simulink model "MicrogridControl"  (R2025b)
settings: Solver=VariableStepAuto  StartTime=0.0  StopTime=8  FixedStep=Ts  RelTol=1e-3
PreLoadFcn:
  | NormalOperation;
  | MicrogridControlParam;
undefined symbols (not defined in the file): base, bessModeInitial, bessSystem, bessVoltage, breakerStatus, DiscIntNeverNeededParam, ee_sli_rtmsupport, event, gcbh, generator, gflInverter, gfmInverter, Inertia, lineInductance, lineResistance, machine, plannedIsland, pmsm, powerLimit, powerQuality, PV, PVInverter, ref, resync, solar, solarInsolationChange, systemFrequency, Ts, windController, windSystem, windTurbine
libraries: nesl_utility x234, ee_lib x174, fl_lib x143, eeGeneralControl x137, simulink x78, eeTransforms x47, slpidlib x23, nesl_utility_internal x12, eePwmGenerator x9, eeSinusoidalMeasurementV2 x9, custom_lib x7, batteryecm_lib x6
(part 7 of 25)

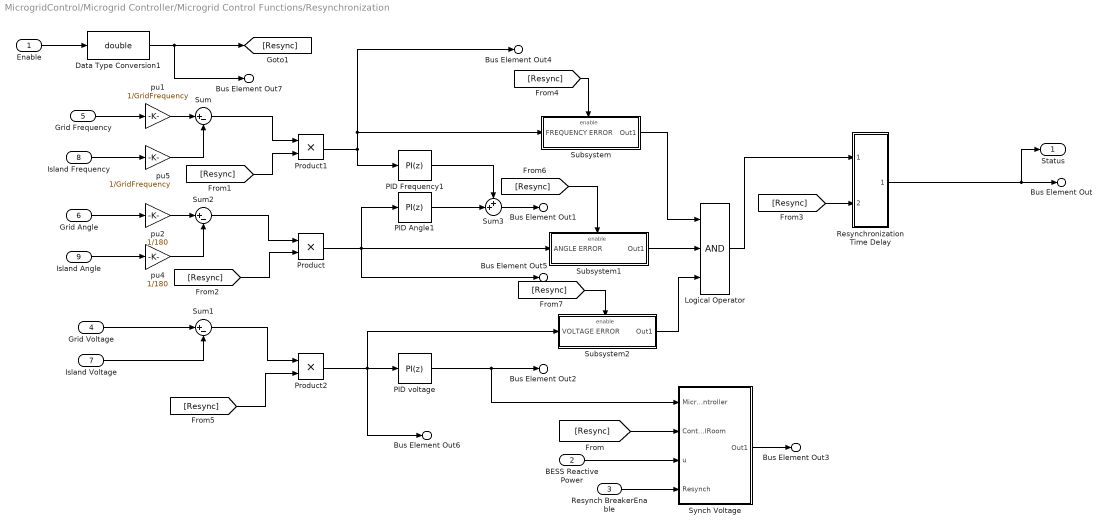
== system MicrogridControl/Microgrid Controller/Microgrid Control Functions/Resynchronization ==
  Enable : Inport
  BESS Reactive Power : Inport  Port=2
  Resynch BreakerEnable : Inport  Port=3
  Grid Voltage : Inport  Port=4
  Grid Frequency : Inport  Port=5
  Grid Angle : Inport  Port=6
  Island Voltage : Inport  Port=7
  Island Frequency : Inport  Port=8
  Island Angle : Inport  Port=9
  Data Type Conversion1 : DataTypeConversion  OutDataTypeStr=double  SaturateOnIntegerOverflow=off  RndMeth=Floor
  Logical Operator : Logic  Inputs=3  AllPortsSameDT=off  OutDataTypeStr=boolean
  PID Angle1 : slpidlib/PID Controller  Controller=PI  Form=Parallel  TimeDomain=Discrete-time  UseExternalTs=off  SampleTime=Ts  IntegratorMethod=Forward Euler  FilterMethod=Forward Euler  ControllerParametersSource=internal  P=KpAngResynch  I=KiAngResynch  UseKiTs=off  D=0  UseExternalDerivativeSource=off  N=100  UseFilter=on  TunerSelectOption=Frequency Response Based  InitialConditionSource=internal  InitialConditionForIntegrator=0  InitialConditionForFilter=0  DifferentiatorICPrevScaledInput=0  ExternalReset=none  TrackingMode=off  Kt=1  LimitOutput=off  SatLimitsSource=internal  UpperSaturationLimit=0.5  LowerSaturationLimit=-0.5  LinearizeAsGain=on  AntiWindupMode=clamping  Kb=1  LimitIntegrator=off  UpperIntegratorSaturationLimit=inf  LowerIntegratorSaturationLimit=-inf  POutMin=[]  POutMax=[]  IOutMin=[]  IOutMax=[]  DOutMin=[]  DOutMax=[]  NOutMin=[]  NOutMax=[]  SumOutMin=[]  SumOutMax=[]  SaturationOutMin=[]  SaturationOutMax=[]  PParamMin=[]  PParamMax=[]  IParamMin=[]  IParamMax=[]  DParamMin=[]  DParamMax=[]  NParamMin=[]  NParamMax=[]  KbParamMin=[]  KbParamMax=[]  KtParamMin=[]  KtParamMax=[]  KbOutMin=[]  KbOutMax=[]  KtOutMin=[]  KtOutMax=[]  IntegratorOutMin=[]  IntegratorOutMax=[]  FilterOutMin=[]  FilterOutMax=[]  SumI1OutMin=[]  SumI1OutMax=[]  SumI2OutMin=[]  SumI2OutMax=[]  SumI3OutMin=[]  SumI3OutMax=[]  SumI4OutMin=[]  SumI4OutMax=[]  SumDOutMin=[]  SumDOutMax=[]  DifferentiatorOutMin=[]  DifferentiatorOutMax=[]  FilterDiffOutCoefMin=[]  FilterDiffOutCoefMax=[]  ReciprocalOutMin=[]  ReciprocalOutMax=[]  SumDenOutMin=[]  SumDenOutMax=[]  SumNumOutMin=[]  SumNumOutMax=[]  DivideOutMin=[]  DivideOutMax=[]  UdiffTsProdOutMin=[]  UdiffTsProdOutMax=[]  NTsProdOutMin=[]  NTsProdOutMax=[]  UintegralTsProdOutMin=[]  UintegralTsProdOutMax=[]  UngainTsProdOutMin=[]  UngainTsProdOutMax=[]  ClampingZeroOutDataTypeStr=Inherit: Inherit via back propagation  ClampingZeroOutMin=[]  ClampingZeroOutMax=[]  FilterDenConstantOutDataTypeStr=Inherit: Inherit via back propagation  FilterDenConstantOutMin=[]  FilterDenConstantOutMax=[]  PCopyOutDataTypeStr=Inherit: Inherit via back propagation  PCopyOutMin=[]  PCopyOutMax=[]  NCopyOutDataTypeStr=Inherit: Inherit via back propagation  NCopyOutMin=[]  NCopyOutMax=[]  IntegratorContinuousStateAttributes=''  IntegratorStateMustResolveToSignalObject=off  IntegratorRTWStateStorageClass=Auto  FilterContinuousStateAttributes=''  FilterStateMustResolveToSignalObject=off  FilterRTWStateStorageClass=Auto  ParallelPVariant=InternalParameters  IdealPVariant=Disabled  IVariant=InternalParameters  DVariant=Disabled  IntegratorVariant=Discrete  SatVariant=Disabled  AWVariant=Passthrough  PCopyVariant=Disabled  TRVariant=Disabled  FdbkBlocksVariant=Forward  IdealPFdbkVariant=Disabled  SatFdbkVariant=Disabled  DerivativeFilterVariant=Disabled  NVariant=Disabled  NCopyVariant=Disabled_SignalSpec  FilterICVariant=Disabled  IntegratorICVariant=InternalICs  ExternalResetVariant=Disabled  TRSumVariant=Passthrough  SumFdbkVariant=Disabled  SumVariant=Sum_PI  TsampFilterVariant=InternalTs  TsampNgainVariant=Passthrough  TsampIntegralVariant=Disabled_SignalSpec  ExternalSaturationOutDataTypeStr=Inherit: Same as second input  DerivativeSourceVariant=Disabled  PreIntVariant=InternalPreInt
  PID Frequency1 : slpidlib/PID Controller  Controller=PI  Form=Parallel  TimeDomain=Discrete-time  UseExternalTs=off  SampleTime=Ts  IntegratorMethod=Forward Euler  FilterMethod=Forward Euler  ControllerParametersSource=internal  P=KpFreResynch  I=KiFreResynch  UseKiTs=off  D=0  UseExternalDerivativeSource=off  N=100  UseFilter=on  TunerSelectOption=Frequency Response Based  InitialConditionSource=internal  InitialConditionForIntegrator=0  InitialConditionForFilter=0  DifferentiatorICPrevScaledInput=0  ExternalReset=none  TrackingMode=off  Kt=1  LimitOutput=off  SatLimitsSource=internal  UpperSaturationLimit=0.05  LowerSaturationLimit=-0.05  LinearizeAsGain=on  AntiWindupMode=clamping  Kb=1  LimitIntegrator=off  UpperIntegratorSaturationLimit=inf  LowerIntegratorSaturationLimit=-inf  POutMin=[]  POutMax=[]  IOutMin=[]  IOutMax=[]  DOutMin=[]  DOutMax=[]  NOutMin=[]  NOutMax=[]  SumOutMin=[]  SumOutMax=[]  SaturationOutMin=[]  SaturationOutMax=[]  PParamMin=[]  PParamMax=[]  IParamMin=[]  IParamMax=[]  DParamMin=[]  DParamMax=[]  NParamMin=[]  NParamMax=[]  KbParamMin=[]  KbParamMax=[]  KtParamMin=[]  KtParamMax=[]  KbOutMin=[]  KbOutMax=[]  KtOutMin=[]  KtOutMax=[]  IntegratorOutMin=[]  IntegratorOutMax=[]  FilterOutMin=[]  FilterOutMax=[]  SumI1OutMin=[]  SumI1OutMax=[]  SumI2OutMin=[]  SumI2OutMax=[]  SumI3OutMin=[]  SumI3OutMax=[]  SumI4OutMin=[]  SumI4OutMax=[]  SumDOutMin=[]  SumDOutMax=[]  DifferentiatorOutMin=[]  DifferentiatorOutMax=[]  FilterDiffOutCoefMin=[]  FilterDiffOutCoefMax=[]  ReciprocalOutMin=[]  ReciprocalOutMax=[]  SumDenOutMin=[]  SumDenOutMax=[]  SumNumOutMin=[]  SumNumOutMax=[]  DivideOutMin=[]  DivideOutMax=[]  UdiffTsProdOutMin=[]  UdiffTsProdOutMax=[]  NTsProdOutMin=[]  NTsProdOutMax=[]  UintegralTsProdOutMin=[]  UintegralTsProdOutMax=[]  UngainTsProdOutMin=[]  UngainTsProdOutMax=[]  ClampingZeroOutDataTypeStr=Inherit: Inherit via back propagation  ClampingZeroOutMin=[]  ClampingZeroOutMax=[]  FilterDenConstantOutDataTypeStr=Inherit: Inherit via back propagation  FilterDenConstantOutMin=[]  FilterDenConstantOutMax=[]  PCopyOutDataTypeStr=Inherit: Inherit via back propagation  PCopyOutMin=[]  PCopyOutMax=[]  NCopyOutDataTypeStr=Inherit: Inherit via back propagation  NCopyOutMin=[]  NCopyOutMax=[]  IntegratorContinuousStateAttributes=''  IntegratorStateMustResolveToSignalObject=off  IntegratorRTWStateStorageClass=Auto  FilterContinuousStateAttributes=''  FilterStateMustResolveToSignalObject=off  FilterRTWStateStorageClass=Auto  ParallelPVariant=InternalParameters  IdealPVariant=Disabled  IVariant=InternalParameters  DVariant=Disabled  IntegratorVariant=Discrete  SatVariant=Disabled  AWVariant=Passthrough  PCopyVariant=Disabled  TRVariant=Disabled  FdbkBlocksVariant=Forward  IdealPFdbkVariant=Disabled  SatFdbkVariant=Disabled  DerivativeFilterVariant=Disabled  NVariant=Disabled  NCopyVariant=Disabled_SignalSpec  FilterICVariant=Disabled  IntegratorICVariant=InternalICs  ExternalResetVariant=Disabled  TRSumVariant=Passthrough  SumFdbkVariant=Disabled  SumVariant=Sum_PI  TsampFilterVariant=InternalTs  TsampNgainVariant=Passthrough  TsampIntegralVariant=Disabled_SignalSpec  ExternalSaturationOutDataTypeStr=Inherit: Same as second input  DerivativeSourceVariant=Disabled  PreIntVariant=InternalPreInt
  PID voltage : slpidlib/PID Controller  Controller=PI  Form=Parallel  TimeDomain=Discrete-time  UseExternalTs=off  SampleTime=Ts  IntegratorMethod=Forward Euler  FilterMethod=Forward Euler  ControllerParametersSource=internal  P=KpVolResynch  I=KiVolResynch  UseKiTs=off  D=0  UseExternalDerivativeSource=off  N=100  UseFilter=on  TunerSelectOption=Frequency Response Based  InitialConditionSource=internal  InitialConditionForIntegrator=1  InitialConditionForFilter=0  DifferentiatorICPrevScaledInput=0  ExternalReset=none  TrackingMode=off  Kt=1  LimitOutput=off  SatLimitsSource=internal  UpperSaturationLimit=1.5  LowerSaturationLimit=-0.05  LinearizeAsGain=on  AntiWindupMode=clamping  Kb=1  LimitIntegrator=off  UpperIntegratorSaturationLimit=inf  LowerIntegratorSaturationLimit=-inf  POutMin=[]  POutMax=[]  IOutMin=[]  IOutMax=[]  DOutMin=[]  DOutMax=[]  NOutMin=[]  NOutMax=[]  SumOutMin=[]  SumOutMax=[]  SaturationOutMin=[]  SaturationOutMax=[]  PParamMin=[]  PParamMax=[]  IParamMin=[]  IParamMax=[]  DParamMin=[]  DParamMax=[]  NParamMin=[]  NParamMax=[]  KbParamMin=[]  KbParamMax=[]  KtParamMin=[]  KtParamMax=[]  KbOutMin=[]  KbOutMax=[]  KtOutMin=[]  KtOutMax=[]  IntegratorOutMin=[]  IntegratorOutMax=[]  FilterOutMin=[]  FilterOutMax=[]  SumI1OutMin=[]  SumI1OutMax=[]  SumI2OutMin=[]  SumI2OutMax=[]  SumI3OutMin=[]  SumI3OutMax=[]  SumI4OutMin=[]  SumI4OutMax=[]  SumDOutMin=[]  SumDOutMax=[]  DifferentiatorOutMin=[]  DifferentiatorOutMax=[]  FilterDiffOutCoefMin=[]  FilterDiffOutCoefMax=[]  ReciprocalOutMin=[]  ReciprocalOutMax=[]  SumDenOutMin=[]  SumDenOutMax=[]  SumNumOutMin=[]  SumNumOutMax=[]  DivideOutMin=[]  DivideOutMax=[]  UdiffTsProdOutMin=[]  UdiffTsProdOutMax=[]  NTsProdOutMin=[]  NTsProdOutMax=[]  UintegralTsProdOutMin=[]  UintegralTsProdOutMax=[]  UngainTsProdOutMin=[]  UngainTsProdOutMax=[]  ClampingZeroOutDataTypeStr=Inherit: Inherit via back propagation  ClampingZeroOutMin=[]  ClampingZeroOutMax=[]  FilterDenConstantOutDataTypeStr=Inherit: Inherit via back propagation  FilterDenConstantOutMin=[]  FilterDenConstantOutMax=[]  PCopyOutDataTypeStr=Inherit: Inherit via back propagation  PCopyOutMin=[]  PCopyOutMax=[]  NCopyOutDataTypeStr=Inherit: Inherit via back propagation  NCopyOutMin=[]  NCopyOutMax=[]  IntegratorContinuousStateAttributes=''  IntegratorStateMustResolveToSignalObject=off  IntegratorRTWStateStorageClass=Auto  FilterContinuousStateAttributes=''  FilterStateMustResolveToSignalObject=off  FilterRTWStateStorageClass=Auto  ParallelPVariant=InternalParameters  IdealPVariant=Disabled  IVariant=InternalParameters  DVariant=Disabled  IntegratorVariant=Discrete  SatVariant=Disabled  AWVariant=Passthrough  PCopyVariant=Disabled  TRVariant=Disabled  FdbkBlocksVariant=Forward  IdealPFdbkVariant=Disabled  SatFdbkVariant=Disabled  DerivativeFilterVariant=Disabled  NVariant=Disabled  NCopyVariant=Disabled_SignalSpec  FilterICVariant=Disabled  IntegratorICVariant=InternalICs  ExternalResetVariant=Disabled  TRSumVariant=Passthrough  SumFdbkVariant=Disabled  SumVariant=Sum_PI  TsampFilterVariant=InternalTs  TsampNgainVariant=Passthrough  TsampIntegralVariant=Disabled_SignalSpec  ExternalSaturationOutDataTypeStr=Inherit: Same as second input  DerivativeSourceVariant=Disabled  PreIntVariant=InternalPreInt
  Product : Product
  Product1 : Product
  Product2 : Product
  Resynchronization Time Delay : Subsystem
  Subsystem : Subsystem
  Subsystem1 : Subsystem
  Subsystem2 : Subsystem
  Sum : Sum  Inputs=|+-
  Sum1 : Sum  Inputs=|+-
  Sum2 : Sum  Inputs=|+-
  Sum3 : Sum  Inputs=++|
  Synch Voltage : Subsystem
  pu1 : Gain  Gain=1/GridFrequency
  pu2 : Gain  Gain=1/180
  pu4 : Gain  Gain=1/180
  pu5 : Gain  Gain=1/GridFrequency
  Status : Outport
  Bus Element Out : Outport  Port=2  PortName=Resync  Element=status
  Bus Element Out1 : Outport  Port=2  PortName=Resync  Element=synchFrequency
  Bus Element Out2 : Outport  Port=2  PortName=Resync  Element=synchVoltage
  Bus Element Out3 : Outport  Port=2  PortName=Resync  Element=synchVoltagedpr
  Bus Element Out4 : Outport  Port=2  PortName=Resync  Element=frequencyerror
  Bus Element Out5 : Outport  Port=2  PortName=Resync  Element=phasError
  Bus Element Out6 : Outport  Port=2  PortName=Resync  Element=voltageMagError
  Bus Element Out7 : Outport  Port=2  PortName=Resync  Element=enableCommand
  wires:
  PID Frequency1/1 -> Sum3/1
  pu1/1 -> Sum/1
  Resynch BreakerEnable/1 -> Synch Voltage/4(Resynch)
  Island Voltage/1 -> Sum1/2
  Product1/1 -> Bus Element Out4/1, Subsystem/1(FREQUENCY ERROR), PID Frequency1/1
  Sum2/1 -> Product/1
  pu4/1 -> Sum2/2
  BESS Reactive Power/1 -> Synch Voltage/3(u)
  PID Angle1/1 -> Sum3/2
  Island Frequency/1 -> pu5/1
  pu2/1 -> Sum2/1
  Data Type Conversion1/1 -> Bus Element Out7/1, [Resync]
  Product2/1 -> PID voltage/1, Bus Element Out6/1, Subsystem2/1(VOLTAGE ERROR)
  Grid Voltage/1 -> Sum1/1
  Island Angle/1 -> pu4/1
  [Resync] -> Product1/2
  Grid Angle/1 -> pu2/1
  Grid Frequency/1 -> pu1/1
  Product/1 -> Bus Element Out5/1, Subsystem1/1(ANGLE ERROR), PID Angle1/1
  Subsystem/1(Out1) -> Logical Operator/1
  Resynchronization Time Delay/1(MGController) -> Bus Element Out/1, Status/1
  pu5/1 -> Sum/2
  [Resync] -> Product2/2
  [Resync] -> Resynchronization Time Delay/2(In2)
  Logical Operator/1 -> Resynchronization Time Delay/1(In1)
  [Resync] -> Synch Voltage/2(ControlRoom)
  Subsystem2/1(Out1) -> Logical Operator/3
  Subsystem1/1(Out1) -> Logical Operator/2
  [Resync] -> Subsystem2/Enable
  Synch Voltage/1(Out1) -> Bus Element Out3/1
  Sum1/1 -> Product2/1
  Enable/1 -> Data Type Conversion1/1
  Sum3/1 -> Bus Element Out1/1
  Sum/1 -> Product1/1
  PID voltage/1 -> Bus Element Out2/1, Synch Voltage/1(MicrogridController)
  [Resync] -> Subsystem/Enable
  [Resync] -> Product/2
  [Resync] -> Subsystem1/Enable

== system MicrogridControl/Microgrid Controller/Microgrid Supervisory Control/Transition and Dispatch Control/On.Black_Start ==
  blackStartComplete : Inport
  blackStartEnable : Inport  Port=2
  " Demux " : Demux  Outputs=1
  " SFunction " : S-Function  Tag=Stateflow S-Function 8  FunctionName=sf_sfun  PortCounts=[2 3]  SFunctionDeploymentMode=off  EnableBusSupport=off
  " Terminator " : Terminator
  blackStartStatus : Outport
  blackStart : Outport  Port=2
  wires:
  blackStartComplete/1 -> " SFunction "/1
  blackStartEnable/1 -> " SFunction "/2
  " SFunction "/2 -> blackStartStatus/1  "blackStartStatus"
  " SFunction "/3 -> blackStart/1  "blackStart"
  " Demux "/1 -> " Terminator "/1
  " SFunction "/1 -> " Demux "/1

== system MicrogridControl/Microgrid Controller/Microgrid Supervisory Control/Transition and Dispatch Control/On.Planned_Islanding ==
  PlannedIslanding : Inport
  " Demux " : Demux  Outputs=1
  " SFunction " : S-Function  Tag=Stateflow S-Function 18  FunctionName=sf_sfun  PortCounts=[1 6]  SFunctionDeploymentMode=off  EnableBusSupport=off
  " Terminator " : Terminator
  PCC : Outport
  plannedIslanding : Outport  Port=2
  plannedIslandingStatus : Outport  Port=3
  mode : Outport  Port=4
  motorBreaker : Outport  Port=5
  wires:
  PlannedIslanding/1 -> " SFunction "/1
  " SFunction "/2 -> PCC/1  "PCC"
  " SFunction "/3 -> plannedIslanding/1  "plannedIslanding"
  " SFunction "/4 -> plannedIslandingStatus/1  "plannedIslandingStatus"
  " SFunction "/5 -> mode/1  "mode"
  " SFunction "/6 -> motorBreaker/1  "motorBreaker"
  " Demux "/1 -> " Terminator "/1
  " SFunction "/1 -> " Demux "/1

== system MicrogridControl/Microgrid Controller/Microgrid Supervisory Control/Transition and Dispatch Control/On.Resynchronization ==
  Resync : Inport
  " Demux " : Demux  Outputs=1
  " SFunction " : S-Function  Tag=Stateflow S-Function 19  FunctionName=sf_sfun  PortCounts=[1 5]  SFunctionDeploymentMode=off  EnableBusSupport=off
  " Terminator " : Terminator
  PCC : Outport
  resync : Outport  Port=2
  resyncStatus : Outport  Port=3
  mode : Outport  Port=4
  wires:
  Resync/1 -> " SFunction "/1
  " SFunction "/2 -> PCC/1  "PCC"
  " SFunction "/3 -> resync/1  "resync"
  " SFunction "/4 -> resyncStatus/1  "resyncStatus"
  " SFunction "/5 -> mode/1  "mode"
  " Demux "/1 -> " Terminator "/1
  " SFunction "/1 -> " Demux "/1

== system MicrogridControl/Microgrid Controller/Microgrid Supervisory Control/Transition and Dispatch Control/On.Steady_State_Grid_Connected ==
  " Demux " : Demux  Outputs=1
  " Ground " : Ground
  " SFunction " : S-Function  Tag=Stateflow S-Function 20  FunctionName=sf_sfun  PortCounts=[1 3]  SFunctionDeploymentMode=off  EnableBusSupport=off
  " Terminator " : Terminator
  emergencyDispatch : Outport
  mode : Outport  Port=2
  wires:
  " SFunction "/2 -> emergencyDispatch/1  "emergencyDispatch"
  " SFunction "/3 -> mode/1  "mode"
  " Ground "/1 -> " SFunction "/1
  " Demux "/1 -> " Terminator "/1
  " SFunction "/1 -> " Demux "/1

== system MicrogridControl/Microgrid Controller/Microgrid Supervisory Control/Transition and Dispatch Control/On.Steady_State_Islanded ==
  plannedIslandingDispatch : Inport
  " Demux " : Demux  Outputs=1
  " SFunction " : S-Function  Tag=Stateflow S-Function 21  FunctionName=sf_sfun  PortCounts=[1 3]  SFunctionDeploymentMode=off  EnableBusSupport=off
  " Terminator " : Terminator
  emergencyDispatch : Outport
  motorBreaker : Outport  Port=2
  wires:
  plannedIslandingDispatch/1 -> " SFunction "/1
  " SFunction "/2 -> emergencyDispatch/1  "emergencyDispatch"
  " SFunction "/3 -> motorBreaker/1  "motorBreaker"
  " Demux "/1 -> " Terminator "/1
  " SFunction "/1 -> " Demux "/1

== system MicrogridControl/Microgrid Controller/Microgrid Supervisory Control/Transition and Dispatch Control/On.Unplanned_Islanding ==
  " Demux " : Demux  Outputs=1
  " Ground " : Ground
  " SFunction " : S-Function  Tag=Stateflow S-Function 22  FunctionName=sf_sfun  PortCounts=[1 3]  SFunctionDeploymentMode=off  EnableBusSupport=off
  " Terminator " : Terminator
  PCC : Outport
  emergencyDispatch : Outport  Port=2
  wires:
  " SFunction "/2 -> PCC/1  "PCC"
  " SFunction "/3 -> emergencyDispatch/1  "emergencyDispatch"
  " Ground "/1 -> " SFunction "/1
  " Demux "/1 -> " Terminator "/1
  " SFunction "/1 -> " Demux "/1

== system MicrogridControl/Microgrid Controller/Reference Generation/Active and Reactive Powers ==
  Planned Islanding : Inport
  Planned Islanding PRef : Inport  Port=2
  Planned Islanding QRef : Inport  Port=3
  Control Room PRef : Inport  Port=4
  Control Room QRef : Inport  Port=5
  Saturation : Saturate  UpperLimit=1  LowerLimit=-1
  Saturation1 : Saturate  UpperLimit=1  LowerLimit=-1
  Sum : Sum  Inputs=|++
  Sum1 : Sum  Inputs=|++
  Switch : Switch  Criteria=u2 > Threshold  Threshold=0.5  SaturateOnIntegerOverflow=off  InputSameDT=off
  Switch1 : Switch  Criteria=u2 > Threshold  Threshold=0.5  SaturateOnIntegerOverflow=off  InputSameDT=off
  PRef : Outport
  QRef : Outport  Port=2
  wires:
  Saturation1/1 -> QRef/1
  Saturation/1 -> PRef/1
  Switch/1 -> Saturation/1  "Pref"
  Sum/1 -> Switch/1
  Switch1/1 -> Saturation1/1  "Qref"
  Sum1/1 -> Switch1/1
  Control Room PRef/1 -> Switch/3, Sum/2
  Control Room QRef/1 -> Sum1/2, Switch1/3
  Planned Islanding/1 -> Switch1/2, Switch/2
  Planned Islanding PRef/1 -> Sum/1
  Planned Islanding QRef/1 -> Sum1/1

== system MicrogridControl/Microgrid Controller/Reference Generation/Frequency ==
  Reference Island Frequency : Inport
  Resynch Command : Inport  Port=2
  Power command : Inport  Port=3
  Resych Frequency : Inport  Port=4
  Black Start : Inport  Port=5
  Black Start Frequency : Inport  Port=6
  Constant1 : Constant  Value=1%frequencyPLL
  Scope : Scope  NumInputPorts=2
      settings: ActiveDisplayYMinimum=-1  ActiveDisplayYMaximum=1  DataLoggingVariableName=ScopeData2
  Scope1 : Scope  NumInputPorts=3
      settings: ActiveDisplayYMinimum=-1  ActiveDisplayYMaximum=1  DataLoggingVariableName=ScopeData3
  Sum : Sum  Inputs=|++
  Switch : Switch  Criteria=u2 > Threshold  Threshold=0.5  SaturateOnIntegerOverflow=off  InputSameDT=off
  Switch1 : Switch  Criteria=u2 > Threshold  Threshold=0.5  SaturateOnIntegerOverflow=off  InputSameDT=off
  Switch2 : Switch  Criteria=u2 > Threshold  Threshold=0.5  SaturateOnIntegerOverflow=off  InputSameDT=off
  FRef : Outport
  wires:
  Switch2/1 -> Switch1/3
  Resych Frequency/1 -> Sum/1
  Black Start Frequency/1 -> Scope1/3, Switch1/1
  Black Start/1 -> Scope1/1, Switch1/2
  Power command/1 -> Switch2/2
  Reference Island Frequency/1 -> Sum/2, Switch/3
  Sum/1 -> Scope/2, Switch/1
  Constant1/1 -> Switch2/1
  Switch/1 -> Switch2/3
  Resynch Command/1 -> Scope/1, Switch/2
  Switch1/1 -> FRef/1, Scope1/2

== system MicrogridControl/Microgrid Controller/Reference Generation/Voltage ==
  Reference Island Voltage : Inport
  Resynch Voltage : Inport  Port=2
  Resynch Command : Inport  Port=3
  Blackstart Command : Inport  Port=4
  Black Start voltage : Inport  Port=5
  Scope : Scope  NumInputPorts=2
      settings: ActiveDisplayYMinimum=-1  ActiveDisplayYMaximum=1
  Scope1 : Scope  NumInputPorts=2
      settings: ActiveDisplayYMinimum=-1  ActiveDisplayYMaximum=1
  Switch1 : Switch  Criteria=u2 > Threshold  Threshold=0.5  SaturateOnIntegerOverflow=off  InputSameDT=off
  Switch2 : Switch  Criteria=u2 > Threshold  Threshold=0.5  SaturateOnIntegerOverflow=off  InputSameDT=off
  VRef : Outport
  wires:
  Switch2/1 -> Scope1/2, VRef/1
  Switch1/1 -> Switch2/3
  Reference Island Voltage/1 -> Scope/1, Switch1/3
  Blackstart Command/1 -> Scope1/1, Switch2/2
  Black Start voltage/1 -> Switch2/1
  Resynch Voltage/1 -> Switch1/1
  Resynch Command/1 -> Scope/2, Switch1/2

== system MicrogridControl/Microgrid Controller/Subsystem1/PLL ==
  abc : Inport
  Frequency Measurement : Subsystem
  Gain : Gain  Gain=1/sqrt(2)
  "Sinusoidal Measurement (PLL, Three-Phase)" : eeSinusoidalMeasurement/Sinusoidal Measurement (PLL, Three-Phase)  Kp_LF=40  Ki_LF=1000  F0=50  Theta0=0  Ts=-1
  Subsystem : Subsystem
  fre : Outport
  angle : Outport  Port=2
  mag : Outport  Port=3
  wires:
  abc/1 -> Frequency Measurement/1(Vabc), "Sinusoidal Measurement (PLL, Three-Phase)"/1
  "Sinusoidal Measurement (PLL, Three-Phase)"/3 -> Gain/1
  "Sinusoidal Measurement (PLL, Three-Phase)"/2 -> Subsystem/1(In)
  Subsystem/1(Out) -> angle/1
  Gain/1 -> mag/1
  Frequency Measurement/1(freq) -> fre/1

== system MicrogridControl/Microgrid Controller/Subsystem1/PLL start at 0.2 s ==
  PCC measurement : Inport
  Constant : Constant  Value=0
  Step : Step  Time=0.2  SampleTime=Ts
  Switch : Switch  Criteria=u2 > Threshold  Threshold=0.5  SaturateOnIntegerOverflow=off  InputSameDT=off
  Out1 : Outport
  wires:
  PCC measurement/1 -> Switch/1
  Switch/1 -> Out1/1
  Constant/1 -> Switch/3
  Step/1 -> Switch/2

== system MicrogridControl/Microgrid Controller/Subsystem1/PLL starts at 0.2 s ==
  PCC measurement : Inport
  Constant1 : Constant  Value=0
  Step : Step  Time=0.2  SampleTime=Ts
  Switch : Switch  Criteria=u2 > Threshold  Threshold=0.5  SaturateOnIntegerOverflow=off  InputSameDT=off
  abc : Outport
  wires:
  PCC measurement/1 -> Switch/1
  Constant1/1 -> Switch/3
  Switch/1 -> abc/1
  Step/1 -> Switch/2

== system MicrogridControl/Microgrid Controller/Subsystem1/PLL1 ==
  abc : Inport
  Frequency Measurement : Subsystem
  Gain : Gain  Gain=1/sqrt(2)
  "Sinusoidal Measurement (PLL, Three-Phase)" : eeSinusoidalMeasurement/Sinusoidal Measurement (PLL, Three-Phase)  Kp_LF=40  Ki_LF=1000  F0=50  Theta0=0  Ts=-1
  Subsystem : Subsystem
  fre : Outport
  angle : Outport  Port=2
  mag : Outport  Port=3
  wires:
  abc/1 -> Frequency Measurement/1(Vabc), "Sinusoidal Measurement (PLL, Three-Phase)"/1
  "Sinusoidal Measurement (PLL, Three-Phase)"/3 -> Gain/1
  "Sinusoidal Measurement (PLL, Three-Phase)"/2 -> Subsystem/1(In)
  Subsystem/1(Out) -> angle/1
  Gain/1 -> mag/1
  Frequency Measurement/1(freq) -> fre/1

== system MicrogridControl/Motor Load/Motor Loads/Subsystem ==
  Gain : Gain  Commented=on  Gain=60/(2*pi)
  Ideal Rotational Motion Sensor : fl_lib/Mechanical/Mechanical Sensors/Ideal Rotational Motion Sensor  Commented=on  reference=foundation.enum.MeasurementReference.difference  acceleration_port=false  velocity_port=true  position_port=false  wrap_angle=false  offset=0 rad
      settings: InternalSimscapePortConfiguration="{\"Bottom\":[],\"Left\":[{\"id\":\"R\",\"label\":\"R\",\"type\":\"foundation.mechanical.rotational.rotational\"}],\"Right\":[{\"id\":\"C\",\"label\":\"C\",\"type\":\"foundation.mechanical.rotational.rotational\"},{\"id\":\"W\",\"label\":\"W\",\"type\":\"output\"}],\"Top\":[]}"
  Ideal Torque Source : fl_lib/Mechanical/Mechanical Sources/Ideal Torque Source
  Mechanical Rotational Reference : fl_lib/Mechanical/Rotational Elements/Mechanical Rotational Reference
  PS Constant : fl_lib/Physical Signals/Sources/PS Constant  Commented=on  constant=300000
  PS Step : fl_lib/Physical Signals/Sources/PS Step  step_time=0.1 s  initial_value=0  final_value=-9000
  PS-Simulink Converter : nesl_utility/PS-Simulink Converter  Commented=on  PhysicalDomain=network_engine_domain  SubClassName=ps_output  LeftPortType=input  RightPortType=output  PseudoPeriodic=off  Frequencies=[]  VectorFormat=inherit  Unit=inherit  AffineConversion=off
  Rotational Friction : fl_lib/Mechanical/Rotational Elements/Rotational Friction  brkwy_trq=25 N*m  brkwy_vel=0.1 rad/s  Col_trq=20 N*m  visc_coef=0.001 N*m*s/rad  w_specify=on  w_priority=None  w=0 rad/s  w_nominal_specify=off  w_nominal_value=1  w_nominal_unit=rad/s  t_specify=on  t_priority=None  t=0 N*m  t_nominal_specify=off  t_nominal_value=1  t_nominal_unit=N*m
  Scope : Scope  Commented=on
      settings: ActiveDisplayYMinimum=566.67789  ActiveDisplayYMaximum=1937.03579
  Step : Step  Commented=on  Time=0.05  After=300000  SampleTime=0
  Conn1 : PMIOPort  Side=Left
  Conn2 : PMIOPort  Port=2  Side=Left
  wires:
  Gain/1 -> Scope/1
  PS-Simulink Converter/1 -> Gain/1
  connections:
  Rotational Friction/RConn1 -- Ideal Rotational Motion Sensor/RConn1 -- Conn2/RConn1 -- Mechanical Rotational Reference/LConn1 -- Ideal Torque Source/RConn2
  Rotational Friction/LConn1 -- Conn1/RConn1 -- Ideal Rotational Motion Sensor/LConn1 -- Ideal Torque Source/LConn1
  PS-Simulink Converter/LConn1 -- Ideal Rotational Motion Sensor/RConn2
  PS Step/RConn1 -- Ideal Torque Source/RConn1

== system MicrogridControl/Solar/Solar Plant Integrated/Detailed ==
  Ir : Inport
  T : Inport  Port=2
  Pref : Inport  Port=3
  Qref : Inport  Port=4
  Mode : Inport  Port=5
  L Filter2 : ee_lib/Passive/RLC Assemblies/RLC (Three-Phase)  port_option=ee.enum.threePhasePort.composite  component_structure=ee.enum.rlc.structure.SeriesRL  R=filterResistance Ohm  L=filterInductance H  C=1e-6 F  R_parasitic=0 Ohm  G_parasitic=0 1/Ohm  IL_specify=on  IL_priority=None  IL=[0, 0, 0] A  IL_nominal_specify=off  IL_nominal_value=1  IL_nominal_unit=A  VC_specify=off  VC_priority=High  VC=[0, 0, 0] V  VC_nominal_specify=off  VC_nominal_value=1  VC_nominal_unit=V
      settings: InternalSimscapePortConfiguration="{\"Bottom\":[],\"Left\":[{\"id\":\"N1\",\"label\":\"~1\",\"type\":\"foundation.electrical.three_phase\"}],\"Right\":[{\"id\":\"N2\",\"label\":\"~2\",\"type\":\"foundation.electrical.three_phase\"}],\"Top\":[]}"
  Measurements : Subsystem
  PV Plant & Controller : Subsystem
  Terminator : Terminator
  ~ : PMIOPort  Side=Right
  Out Bus Element23 : Outport  PortName=Meas  Element=activePower
  Out Bus Element1 : Outport  PortName=Meas  Element=reactivePower
  Out Bus Element2 : Outport  PortName=Meas  Element=voltage
  Out Bus Element3 : Outport  PortName=Meas  Element=current
  wires:
  Measurements/2(Q) -> Out Bus Element1/1
  Measurements/4(I) -> Out Bus Element3/1, PV Plant & Controller/5(Iabc)
  Qref/1 -> PV Plant & Controller/3(Qref)
  Ir/1 -> PV Plant & Controller/1(Insolation)
  Measurements/3(V) -> Out Bus Element2/1, PV Plant & Controller/4(Vabc)
  Measurements/1(P) -> Out Bus Element23/1
  T/1 -> Terminator/1
  Pref/1 -> PV Plant & Controller/2(Pref)
  Mode/1 -> PV Plant & Controller/6(Mode)
  connections:
  L Filter2/RConn1 -- Measurements/LConn1
  L Filter2/LConn1 -- PV Plant & Controller/RConn1
  Measurements/RConn1 -- ~/RConn1

== system MicrogridControl/Solar/Solar Plant Integrated/Simplified ==
  Ir : Inport
  T : Inport  Port=2
  Pref : Inport  Port=3
  Qref : Inport  Port=4
  Mode : Inport  Port=5
  Measurements : Subsystem
  Simulink-PS Converter{,1..4} (5 alike) : nesl_utility/Simulink-PS Converter  PhysicalDomain=network_engine_domain  SubClassName=ps_input  LeftPortType=input  RightPortType=output  PseudoPeriodic=off  Frequencies=[]  NoiseDistribution=none  NoiseParameters=[]  Unit=1  AffineConversion=off  FilteringAndDerivatives=provide  SimscapeFilterOrder=1  InputFilterTimeConstant=0.001  UdotUserProvided=0
  solar_plant : custom_lib/solar_plant  port_option=ee.enum.threePhasePort.composite  FRated=frequency Hz  VRated=Vac V  PlantRating=plantRating kW  modelling_option=ModellingOption.powerReference  Vdc=2*Vac*sqrt(2/3) V  IMaxPU=iMaxPU  efficiency=efficiency  IrRef=irradianceSTC W/m^2  T=temperatureSTC K  PVTech=PanelTechnology.polycrystallinePanel  PanelRating=panelRating W  VocRef=Voc V  IscRef=Isc A  alpha=alpha 1/K  beta=beta 1/K  delta=0.111
      settings: InternalSimscapePortConfiguration="{\"Bottom\":[],\"Left\":[{\"id\":\"Ir\",\"label\":\"Ir\",\"type\":\"input\"},{\"id\":\"Tsim\",\"label\":\"T\",\"type\":\"input\"},{\"id\":\"Mode\",\"label\":\"Mode\",\"type\":\"input\"},{\"id\":\"Pref\",\"label\":\"Pref\",\"type\":\"input\"},{\"id\":\"Qref\",\"label\":\"Qref\",\"type\":\"input\"}],\"Right\":[{\"id\":\"N\",\"label\":\"~\",\"type\":\"foundation.electrical.three_phase\"},{\"id\":\"l\",\"label\":\"l\",\"type\":\"output\"},{\"id\":\"p\",\"label\":\"p\",\"type\":\"output\"}],\"Top\":[]}"
  ~ : PMIOPort  Side=Right
  Bus Element Out : Outport  PortName=Meas  Element=activePower
  BusElementOut : Outport  PortName=Meas  Element=reactivePower
  BusElementOut1 : Outport  PortName=Meas  Element=voltage
  BusElementOut2 : Outport  PortName=Meas  Element=current
  wires:
  Measurements/4(I) -> BusElementOut2/1
  Measurements/3(V) -> BusElementOut1/1
  Measurements/2(Q) -> BusElementOut/1
  Measurements/1(P) -> Bus Element Out/1
  Ir/1 -> Simulink-PS Converter/1
  T/1 -> Simulink-PS Converter1/1
  Pref/1 -> Simulink-PS Converter2/1
  Qref/1 -> Simulink-PS Converter3/1
  Mode/1 -> Simulink-PS Converter4/1
  connections:
  solar_plant/LConn5 -- Simulink-PS Converter3/RConn1
  solar_plant/LConn3 -- Simulink-PS Converter4/RConn1
  ~/RConn1 -- Measurements/RConn1
  Measurements/LConn1 -- solar_plant/RConn1
  Simulink-PS Converter/RConn1 -- solar_plant/LConn1
  Simulink-PS Converter1/RConn1 -- solar_plant/LConn2
  solar_plant/LConn4 -- Simulink-PS Converter2/RConn1

== system MicrogridControl/Solar/Solar Plant Integrated1/Detailed ==
  Ir : Inport
  T : Inport  Port=2
  Pref : Inport  Port=3
  Qref : Inport  Port=4
  Mode : Inport  Port=5
  L Filter2 : ee_lib/Passive/RLC Assemblies/RLC (Three-Phase)  port_option=ee.enum.threePhasePort.composite  component_structure=ee.enum.rlc.structure.SeriesRL  R=filterResistance Ohm  L=filterInductance H  C=1e-6 F  R_parasitic=0 Ohm  G_parasitic=0 1/Ohm  IL_specify=on  IL_priority=None  IL=[0, 0, 0] A  IL_nominal_specify=off  IL_nominal_value=1  IL_nominal_unit=A  VC_specify=off  VC_priority=High  VC=[0, 0, 0] V  VC_nominal_specify=off  VC_nominal_value=1  VC_nominal_unit=V
      settings: InternalSimscapePortConfiguration="{\"Bottom\":[],\"Left\":[{\"id\":\"N1\",\"label\":\"~1\",\"type\":\"foundation.electrical.three_phase\"}],\"Right\":[{\"id\":\"N2\",\"label\":\"~2\",\"type\":\"foundation.electrical.three_phase\"}],\"Top\":[]}"
  Measurements : Subsystem
  PV Plant & Controller : Subsystem
  Terminator : Terminator
  ~ : PMIOPort  Side=Right
  Out Bus Element23 : Outport  PortName=Meas  Element=activePower
  Out Bus Element1 : Outport  PortName=Meas  Element=reactivePower
  Out Bus Element2 : Outport  PortName=Meas  Element=voltage
  Out Bus Element3 : Outport  PortName=Meas  Element=current
  wires:
  Measurements/2(Q) -> Out Bus Element1/1
  Measurements/4(I) -> Out Bus Element3/1, PV Plant & Controller/5(Iabc)
  Qref/1 -> PV Plant & Controller/3(Qref)
  Ir/1 -> PV Plant & Controller/1(Insolation)
  Measurements/3(V) -> Out Bus Element2/1, PV Plant & Controller/4(Vabc)
  Measurements/1(P) -> Out Bus Element23/1
  T/1 -> Terminator/1
  Pref/1 -> PV Plant & Controller/2(Pref)
  Mode/1 -> PV Plant & Controller/6(Mode)
  connections:
  L Filter2/RConn1 -- Measurements/LConn1
  L Filter2/LConn1 -- PV Plant & Controller/RConn1
  Measurements/RConn1 -- ~/RConn1

== system MicrogridControl/Solar/Solar Plant Integrated1/Simplified ==
  Ir : Inport
  T : Inport  Port=2
  Pref : Inport  Port=3
  Qref : Inport  Port=4
  Mode : Inport  Port=5
  Measurements : Subsystem
  Simulink-PS Converter{,1..4} (5 alike) : nesl_utility/Simulink-PS Converter  PhysicalDomain=network_engine_domain  SubClassName=ps_input  LeftPortType=input  RightPortType=output  PseudoPeriodic=off  Frequencies=[]  NoiseDistribution=none  NoiseParameters=[]  Unit=1  AffineConversion=off  FilteringAndDerivatives=provide  SimscapeFilterOrder=1  InputFilterTimeConstant=0.001  UdotUserProvided=0
  solar_plant : custom_lib/solar_plant  port_option=ee.enum.threePhasePort.composite  FRated=frequency Hz  VRated=Vac V  PlantRating=plantRating kW  modelling_option=ModellingOption.powerReference  Vdc=2*Vac*sqrt(2/3) V  IMaxPU=iMaxPU  efficiency=efficiency  IrRef=irradianceSTC W/m^2  T=temperatureSTC K  PVTech=PanelTechnology.polycrystallinePanel  PanelRating=panelRating W  VocRef=Voc V  IscRef=Isc A  alpha=alpha 1/K  beta=beta 1/K  delta=0.111
      settings: InternalSimscapePortConfiguration="{\"Bottom\":[],\"Left\":[{\"id\":\"Ir\",\"label\":\"Ir\",\"type\":\"input\"},{\"id\":\"Tsim\",\"label\":\"T\",\"type\":\"input\"},{\"id\":\"Mode\",\"label\":\"Mode\",\"type\":\"input\"},{\"id\":\"Pref\",\"label\":\"Pref\",\"type\":\"input\"},{\"id\":\"Qref\",\"label\":\"Qref\",\"type\":\"input\"}],\"Right\":[{\"id\":\"N\",\"label\":\"~\",\"type\":\"foundation.electrical.three_phase\"},{\"id\":\"l\",\"label\":\"l\",\"type\":\"output\"},{\"id\":\"p\",\"label\":\"p\",\"type\":\"output\"}],\"Top\":[]}"
  ~ : PMIOPort  Side=Right
  Bus Element Out : Outport  PortName=Meas  Element=activePower
  BusElementOut : Outport  PortName=Meas  Element=reactivePower
  BusElementOut1 : Outport  PortName=Meas  Element=voltage
  BusElementOut2 : Outport  PortName=Meas  Element=current
  wires:
  Measurements/4(I) -> BusElementOut2/1
  Measurements/3(V) -> BusElementOut1/1
  Measurements/2(Q) -> BusElementOut/1
  Measurements/1(P) -> Bus Element Out/1
  Ir/1 -> Simulink-PS Converter/1
  T/1 -> Simulink-PS Converter1/1
  Pref/1 -> Simulink-PS Converter2/1
  Qref/1 -> Simulink-PS Converter3/1
  Mode/1 -> Simulink-PS Converter4/1
  connections:
  solar_plant/LConn5 -- Simulink-PS Converter3/RConn1
  solar_plant/LConn3 -- Simulink-PS Converter4/RConn1
  ~/RConn1 -- Measurements/RConn1
  Measurements/LConn1 -- solar_plant/RConn1
  Simulink-PS Converter/RConn1 -- solar_plant/LConn1
  Simulink-PS Converter1/RConn1 -- solar_plant/LConn2
  solar_plant/LConn4 -- Simulink-PS Converter2/RConn1

== system MicrogridControl/Solar/Transformer/Detailed ==
  Two-Winding Transformer (Three-Phase)2 : ee_lib/Passive/Transformers/Two-Winding Transformer (Three-Phase)  SRated=1.5e6 A*V  FRated=systemFrequency Hz  Winding1Connection=ee.enum.windingconnection.Yg  VRated1=690 V  Winding2Connection=ee.enum.windingconnection.Yg  VRated2=11000 V  CoreType=ee.enum.coretype.threelimb  pu_Rw1=0.01  pu_Rw2=0.01  leakage_reactance_option=ee.enum.transformer_leakage.include  pu_Xl1=0.05  pu_Xl2=0.05  magnetizing_resistance_option=ee.enum.transformer_magnetizingResistance.exclude  pu_Rm=500  magnetizing_reactance_option=ee.enum.transformer_magnetizingReactance.exclude  saturation_option=ee.enum.transformer_saturation.exclude  pu_Xm=500  current_data=[0, .002, 1, 2]  magnetic_flux_data=[0, 1.2, 1.5, 1.51]  pu_X0=0.5  i1_specify=off  i1_priority=None  i1=[0, 0, 0] A  i1_nominal_specify=off  i1_nominal_value=1  i1_nominal_unit=A  i2_specify=off  i2_priority=None  i2=[0, 0, 0] A  i2_nominal_specify=off  i2_nominal_value=1  i2_nominal_unit=A  phi_specify=off  phi_priority=None  phi=[0, 0, 0]  phi_nominal_specify=off  phi_nominal_value=1  phi_nominal_unit=1  power_dissipated_specify=off  power_dissipated_priority=None  power_dissipated=0 W  power_dissipated_nominal_specify=off  power_dissipated_nominal_value=1  power_dissipated_nominal_unit=W
      settings: InternalSimscapePortConfiguration="{\"Bottom\":[],\"Left\":[{\"id\":\"N1\",\"label\":\"~1\",\"type\":\"foundation.electrical.three_phase\"}],\"Right\":[{\"id\":\"N2\",\"label\":\"~2\",\"type\":\"foundation.electrical.three_phase\"}],\"Top\":[]}"
  In : PMIOPort  Side=Left
  Out : PMIOPort  Port=2  Side=Right
  connections:
  Two-Winding Transformer (Three-Phase)2/LConn1 -- In/RConn1
  Two-Winding Transformer (Three-Phase)2/RConn1 -- Out/RConn1

== system MicrogridControl/Solar/Transformer/Simplified ==
  Electrical Reference : fl_lib/Electrical/Electrical Elements/Electrical Reference
  Electrical Reference1 : fl_lib/Electrical/Electrical Elements/Electrical Reference
  Ideal Transformer : fl_lib/Electrical/Electrical Elements/Ideal Transformer  n=windingRatio  i1_specify=off  i1_priority=None  i1=0 A  i1_nominal_specify=off  i1_nominal_value=1  i1_nominal_unit=A  v1_specify=off  v1_priority=None  v1=0 V  v1_nominal_specify=off  v1_nominal_value=1  v1_nominal_unit=V  i2_specify=off  i2_priority=None  i2=0 A  i2_nominal_specify=off  i2_nominal_value=1  i2_nominal_unit=A  v2_specify=off  v2_priority=None  v2=0 V  v2_nominal_specify=off  v2_nominal_value=1  v2_nominal_unit=V
  Ideal Transformer1 : fl_lib/Electrical/Electrical Elements/Ideal Transformer  n=windingRatio  i1_specify=off  i1_priority=None  i1=0 A  i1_nominal_specify=off  i1_nominal_value=1  i1_nominal_unit=A  v1_specify=off  v1_priority=None  v1=0 V  v1_nominal_specify=off  v1_nominal_value=1  v1_nominal_unit=V  i2_specify=off  i2_priority=None  i2=0 A  i2_nominal_specify=off  i2_nominal_value=1  i2_nominal_unit=A  v2_specify=off  v2_priority=None  v2=0 V  v2_nominal_specify=off  v2_nominal_value=1  v2_nominal_unit=V
  Ideal Transformer2 : fl_lib/Electrical/Electrical Elements/Ideal Transformer  n=windingRatio  i1_specify=off  i1_priority=None  i1=0 A  i1_nominal_specify=off  i1_nominal_value=1  i1_nominal_unit=A  v1_specify=off  v1_priority=None  v1=0 V  v1_nominal_specify=off  v1_nominal_value=1  v1_nominal_unit=V  i2_specify=off  i2_priority=None  i2=0 A  i2_nominal_specify=off  i2_nominal_value=1  i2_nominal_unit=A  v2_specify=off  v2_priority=None  v2=0 V  v2_nominal_specify=off  v2_nominal_value=1  v2_nominal_unit=V
  Phase Splitter : ee_lib/Connectors & References/Phase Splitter
  Phase Splitter1 : ee_lib/Connectors & References/Phase Splitter
  RLC (Three-Phase) : ee_lib/Passive/RLC Assemblies/RLC (Three-Phase)  Commented=through  port_option=ee.enum.threePhasePort.composite  component_structure=ee.enum.rlc.structure.R  R=1e-9 Ohm  L=1e-3 H  C=1e-6 F  R_parasitic=0 Ohm  G_parasitic=0 1/Ohm  IL_specify=off  IL_priority=High  IL=[0, 0, 0] A  IL_nominal_specify=off  IL_nominal_value=1  IL_nominal_unit=A  VC_specify=off  VC_priority=High  VC=[0, 0, 0] V  VC_nominal_specify=off  VC_nominal_value=1  VC_nominal_unit=V
      settings: InternalSimscapePortConfiguration="{\"Bottom\":[],\"Left\":[{\"id\":\"N1\",\"label\":\"~1\",\"type\":\"foundation.electrical.three_phase\"}],\"Right\":[{\"id\":\"N2\",\"label\":\"~2\",\"type\":\"foundation.electrical.three_phase\"}],\"Top\":[]}"
  In : PMIOPort  Side=Left
  Out : PMIOPort  Port=2  Side=Right
  connections:
  Ideal Transformer/RConn2 -- Electrical Reference1/LConn1 -- Ideal Transformer1/RConn2 -- Ideal Transformer2/RConn2
  Phase Splitter/RConn3 -- Ideal Transformer2/LConn1
  Phase Splitter/RConn2 -- Ideal Transformer1/LConn1
  Phase Splitter/RConn1 -- Ideal Transformer/LConn1
  Ideal Transformer/LConn2 -- Electrical Reference/LConn1 -- Ideal Transformer1/LConn2 -- Ideal Transformer2/LConn2
  Phase Splitter/LConn1 -- In/RConn1
  Phase Splitter1/LConn1 -- RLC (Three-Phase)/LConn1
  Ideal Transformer/RConn1 -- Phase Splitter1/RConn1
  Ideal Transformer2/RConn1 -- Phase Splitter1/RConn3
  Ideal Transformer1/RConn1 -- Phase Splitter1/RConn2
  RLC (Three-Phase)/RConn1 -- Out/RConn1

== system MicrogridControl/Solar/Transformer1/Detailed ==
  Two-Winding Transformer (Three-Phase)2 : ee_lib/Passive/Transformers/Two-Winding Transformer (Three-Phase)  SRated=1.5e6 A*V  FRated=systemFrequency Hz  Winding1Connection=ee.enum.windingconnection.Yg  VRated1=690 V  Winding2Connection=ee.enum.windingconnection.Yg  VRated2=11000 V  CoreType=ee.enum.coretype.threelimb  pu_Rw1=0.01  pu_Rw2=0.01  leakage_reactance_option=ee.enum.transformer_leakage.include  pu_Xl1=0.05  pu_Xl2=0.05  magnetizing_resistance_option=ee.enum.transformer_magnetizingResistance.exclude  pu_Rm=500  magnetizing_reactance_option=ee.enum.transformer_magnetizingReactance.exclude  saturation_option=ee.enum.transformer_saturation.exclude  pu_Xm=500  current_data=[0, .002, 1, 2]  magnetic_flux_data=[0, 1.2, 1.5, 1.51]  pu_X0=0.5  i1_specify=off  i1_priority=None  i1=[0, 0, 0] A  i1_nominal_specify=off  i1_nominal_value=1  i1_nominal_unit=A  i2_specify=off  i2_priority=None  i2=[0, 0, 0] A  i2_nominal_specify=off  i2_nominal_value=1  i2_nominal_unit=A  phi_specify=off  phi_priority=None  phi=[0, 0, 0]  phi_nominal_specify=off  phi_nominal_value=1  phi_nominal_unit=1  power_dissipated_specify=off  power_dissipated_priority=None  power_dissipated=0 W  power_dissipated_nominal_specify=off  power_dissipated_nominal_value=1  power_dissipated_nominal_unit=W
      settings: InternalSimscapePortConfiguration="{\"Bottom\":[],\"Left\":[{\"id\":\"N1\",\"label\":\"~1\",\"type\":\"foundation.electrical.three_phase\"}],\"Right\":[{\"id\":\"N2\",\"label\":\"~2\",\"type\":\"foundation.electrical.three_phase\"}],\"Top\":[]}"
  In : PMIOPort  Side=Left
  Out : PMIOPort  Port=2  Side=Right
  connections:
  Two-Winding Transformer (Three-Phase)2/LConn1 -- In/RConn1
  Two-Winding Transformer (Three-Phase)2/RConn1 -- Out/RConn1

== system MicrogridControl/Solar/Transformer1/Simplified ==
  Electrical Reference : fl_lib/Electrical/Electrical Elements/Electrical Reference
  Electrical Reference1 : fl_lib/Electrical/Electrical Elements/Electrical Reference
  Ideal Transformer : fl_lib/Electrical/Electrical Elements/Ideal Transformer  n=windingRatio  i1_specify=off  i1_priority=None  i1=0 A  i1_nominal_specify=off  i1_nominal_value=1  i1_nominal_unit=A  v1_specify=off  v1_priority=None  v1=0 V  v1_nominal_specify=off  v1_nominal_value=1  v1_nominal_unit=V  i2_specify=off  i2_priority=None  i2=0 A  i2_nominal_specify=off  i2_nominal_value=1  i2_nominal_unit=A  v2_specify=off  v2_priority=None  v2=0 V  v2_nominal_specify=off  v2_nominal_value=1  v2_nominal_unit=V
  Ideal Transformer1 : fl_lib/Electrical/Electrical Elements/Ideal Transformer  n=windingRatio  i1_specify=off  i1_priority=None  i1=0 A  i1_nominal_specify=off  i1_nominal_value=1  i1_nominal_unit=A  v1_specify=off  v1_priority=None  v1=0 V  v1_nominal_specify=off  v1_nominal_value=1  v1_nominal_unit=V  i2_specify=off  i2_priority=None  i2=0 A  i2_nominal_specify=off  i2_nominal_value=1  i2_nominal_unit=A  v2_specify=off  v2_priority=None  v2=0 V  v2_nominal_specify=off  v2_nominal_value=1  v2_nominal_unit=V
  Ideal Transformer2 : fl_lib/Electrical/Electrical Elements/Ideal Transformer  n=windingRatio  i1_specify=off  i1_priority=None  i1=0 A  i1_nominal_specify=off  i1_nominal_value=1  i1_nominal_unit=A  v1_specify=off  v1_priority=None  v1=0 V  v1_nominal_specify=off  v1_nominal_value=1  v1_nominal_unit=V  i2_specify=off  i2_priority=None  i2=0 A  i2_nominal_specify=off  i2_nominal_value=1  i2_nominal_unit=A  v2_specify=off  v2_priority=None  v2=0 V  v2_nominal_specify=off  v2_nominal_value=1  v2_nominal_unit=V
  Phase Splitter : ee_lib/Connectors & References/Phase Splitter
  Phase Splitter1 : ee_lib/Connectors & References/Phase Splitter
  RLC (Three-Phase) : ee_lib/Passive/RLC Assemblies/RLC (Three-Phase)  Commented=through  port_option=ee.enum.threePhasePort.composite  component_structure=ee.enum.rlc.structure.R  R=1e-9 Ohm  L=1e-3 H  C=1e-6 F  R_parasitic=0 Ohm  G_parasitic=0 1/Ohm  IL_specify=off  IL_priority=High  IL=[0, 0, 0] A  IL_nominal_specify=off  IL_nominal_value=1  IL_nominal_unit=A  VC_specify=off  VC_priority=High  VC=[0, 0, 0] V  VC_nominal_specify=off  VC_nominal_value=1  VC_nominal_unit=V
      settings: InternalSimscapePortConfiguration="{\"Bottom\":[],\"Left\":[{\"id\":\"N1\",\"label\":\"~1\",\"type\":\"foundation.electrical.three_phase\"}],\"Right\":[{\"id\":\"N2\",\"label\":\"~2\",\"type\":\"foundation.electrical.three_phase\"}],\"Top\":[]}"
  In : PMIOPort  Side=Left
  Out : PMIOPort  Port=2  Side=Right
  connections:
  Ideal Transformer/RConn2 -- Electrical Reference1/LConn1 -- Ideal Transformer1/RConn2 -- Ideal Transformer2/RConn2
  Phase Splitter/RConn3 -- Ideal Transformer2/LConn1
  Phase Splitter/RConn2 -- Ideal Transformer1/LConn1
  Phase Splitter/RConn1 -- Ideal Transformer/LConn1
  Ideal Transformer/LConn2 -- Electrical Reference/LConn1 -- Ideal Transformer1/LConn2 -- Ideal Transformer2/LConn2
  Phase Splitter/LConn1 -- In/RConn1
  RLC (Three-Phase)/RConn1 -- Out/RConn1
  Ideal Transformer/RConn1 -- Phase Splitter1/RConn1
  Ideal Transformer2/RConn1 -- Phase Splitter1/RConn3
  Ideal Transformer1/RConn1 -- Phase Splitter1/RConn2
  Phase Splitter1/LConn1 -- RLC (Three-Phase)/LConn1

== system MicrogridControl/Subsystem15/Transformer/Detailed ==
  Two-Winding Transformer (Three-Phase) : ee_lib/Passive/Transformers/Two-Winding Transformer (Three-Phase)  SRated=100e6 A*V  FRated=systemFrequency Hz  Winding1Connection=ee.enum.windingconnection.Yg  VRated1=33000 V  Winding2Connection=ee.enum.windingconnection.Yg  VRated2=11000 V  CoreType=ee.enum.coretype.threelimb  pu_Rw1=0.01  pu_Rw2=0.01  leakage_reactance_option=ee.enum.transformer_leakage.include  pu_Xl1=0.05  pu_Xl2=0.05  magnetizing_resistance_option=ee.enum.transformer_magnetizingResistance.exclude  pu_Rm=500  magnetizing_reactance_option=ee.enum.transformer_magnetizingReactance.exclude  saturation_option=ee.enum.transformer_saturation.exclude  pu_Xm=500  current_data=[0, .002, 1, 2]  magnetic_flux_data=[0, 1.2, 1.5, 1.51]  pu_X0=0.5  i1_specify=off  i1_priority=None  i1=[0, 0, 0] A  i1_nominal_specify=off  i1_nominal_value=1  i1_nominal_unit=A  i2_specify=off  i2_priority=None  i2=[0, 0, 0] A  i2_nominal_specify=off  i2_nominal_value=1  i2_nominal_unit=A  phi_specify=off  phi_priority=None  phi=[0, 0, 0]  phi_nominal_specify=off  phi_nominal_value=1  phi_nominal_unit=1  power_dissipated_specify=off  power_dissipated_priority=None  power_dissipated=0 W  power_dissipated_nominal_specify=off  power_dissipated_nominal_value=1  power_dissipated_nominal_unit=W
      settings: InternalSimscapePortConfiguration="{\"Bottom\":[],\"Left\":[{\"id\":\"N1\",\"label\":\"~1\",\"type\":\"foundation.electrical.three_phase\"}],\"Right\":[{\"id\":\"N2\",\"label\":\"~2\",\"type\":\"foundation.electrical.three_phase\"}],\"Top\":[]}"
  In : PMIOPort  Side=Left
  Out : PMIOPort  Port=2  Side=Right
  connections:
  Two-Winding Transformer (Three-Phase)/LConn1 -- In/RConn1
  Two-Winding Transformer (Three-Phase)/RConn1 -- Out/RConn1
